simulink model "main032_StepChange_FH"  (R2023b)
settings: Solver=VariableStepAuto  StartTime=0.0  StopTime=20  RelTol=1e-3
settings Model: Creator=YYlab_05  LastModifiedBy=YYlab_05

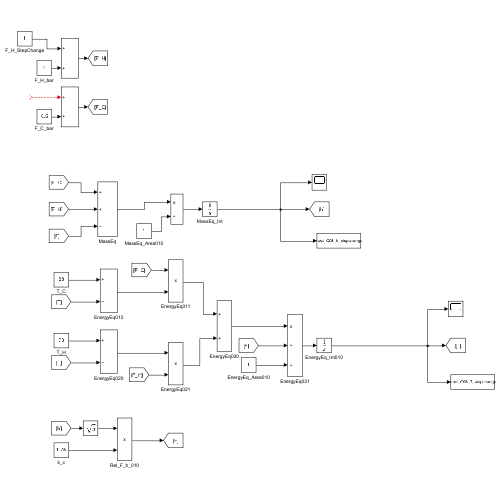
[thumbnail: Simulink's stored preview of the top-level diagram]
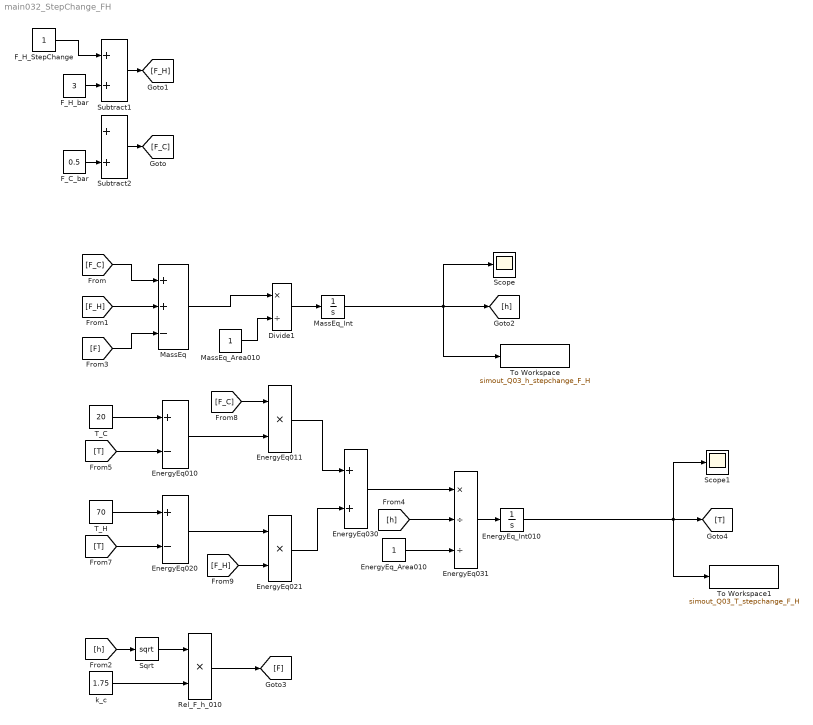
== system main032_StepChange_FH ==
  Divide1 : Product  Inputs=*/
  EnergyEq010 : Sum  Inputs=+-
  EnergyEq011 : Product  Inputs=**
  EnergyEq020 : Sum  Inputs=+-
  EnergyEq021 : Product  Inputs=**
  EnergyEq030 : Sum
  EnergyEq031 : Product  Inputs=*//
  EnergyEq_Area010 : Constant
  EnergyEq_Int010 : Integrator  InitialCondition=(3*70 + 0.5*20)/ (3.5)
  F_C_bar : Constant  Value=0.5
  F_H_StepChange : Constant
  F_H_bar : Constant  Value=3
  MassEq : Sum  Inputs=++-
  MassEq_Area010 : Constant
  MassEq_Int : Integrator  InitialCondition=4
  Rel_F_h_010 : Product  Inputs=**
  Scope : Scope
  Scope1 : Scope
  Sqrt : Sqrt
  Subtract1 : Sum
  Subtract2 : Sum
  T_C : Constant  Value=20
  T_H : Constant  Value=70
  To Workspace : ToWorkspace  VariableName=simout_Q03_h_stepchange_F_H  SaveFormat=Timeseries  SampleTime=-1
  To Workspace1 : ToWorkspace  VariableName=simout_Q03_T_stepchange_F_H  SaveFormat=Timeseries  SampleTime=-1
  k_c : Constant  Value=1.75
  wires:
  Sqrt/1 -> Rel_F_h_010/1
  [h] -> Sqrt/1
  Rel_F_h_010/1 -> [F]
  k_c/1 -> Rel_F_h_010/2
  [F_C] -> MassEq/1
  [F_H] -> MassEq/2
  [F] -> MassEq/3
  MassEq/1 -> Divide1/1
  MassEq_Area010/1 -> Divide1/2
  Divide1/1 -> MassEq_Int/1
  T_C/1 -> EnergyEq010/1
  [T] -> EnergyEq010/2
  T_H/1 -> EnergyEq020/1
  [T] -> EnergyEq020/2
  [F_C] -> EnergyEq011/1
  EnergyEq010/1 -> EnergyEq011/2
  EnergyEq020/1 -> EnergyEq021/1
  [F_H] -> EnergyEq021/2
  EnergyEq011/1 -> EnergyEq030/1
  EnergyEq021/1 -> EnergyEq030/2
  EnergyEq030/1 -> EnergyEq031/1
  [h] -> EnergyEq031/2
  EnergyEq_Area010/1 -> EnergyEq031/3
  EnergyEq031/1 -> EnergyEq_Int010/1
  F_H_bar/1 -> Subtract1/2
  Subtract1/1 -> [F_H]
  F_H_StepChange/1 -> Subtract1/1
  Subtract2/1 -> [F_C]
  ? -> Subtract2/1
  F_C_bar/1 -> Subtract2/2
  MassEq_Int/1 -> To Workspace/1, Scope/1, [h]
  EnergyEq_Int010/1 -> Scope1/1, [T], To Workspace1/1
